simulink model "ESTS_UOD_test"  (R2023b)
settings: Solver=VariableStepAuto  StartTime=0.0  StopTime=10.0  RelTol=1e-3
libraries: ESTS_UOD x1, simulink x1
settings Model: Creator=blatak  LastModifiedBy=blatak

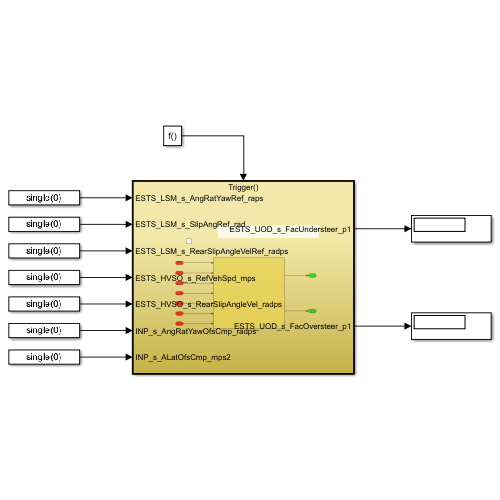
[thumbnail: Simulink's stored preview of the top-level diagram]
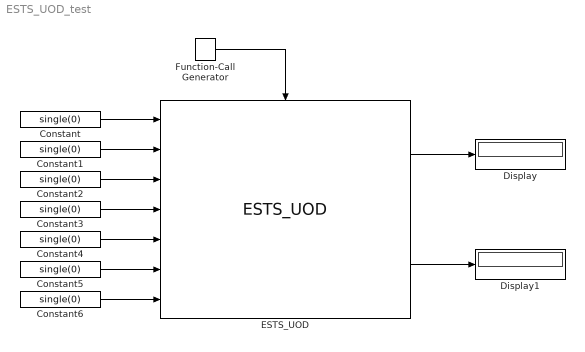
== system ESTS_UOD_test ==
  Constant{,1..6} (7 alike) : Constant  Value=single(0)
  Display : Display
  Display1 : Display
  ESTS_UOD : ESTS_UOD/ESTS_UOD  SystemSampleTime=-1  VariantActivationTime=update diagram  AllowFlexibleInterface=on  Latency=0  AutoFrameSizeCalculation=off
  Function-Call Generator : simulink/Ports & Subsystems/Function-Call Generator  sample_time=0.01  numberOfIterations=1  DisallowWideOutput=off
  wires:
  Function-Call Generator/1 -> ESTS_UOD/Trigger
  Constant/1 -> ESTS_UOD/1
  Constant1/1 -> ESTS_UOD/2
  Constant2/1 -> ESTS_UOD/3
  Constant3/1 -> ESTS_UOD/4
  Constant4/1 -> ESTS_UOD/5
  Constant5/1 -> ESTS_UOD/6
  Constant6/1 -> ESTS_UOD/7
  ESTS_UOD/1 -> Display/1
  ESTS_UOD/2 -> Display1/1
